simulink model "vehicle_ice"  (R2017a)
settings: Solver=FixedStepDiscrete  StartTime=0.0  StopTime=1400  FixedStep=abs(Ts)  RelTol=1e-3
InitFcn:
  | if ~exist('Ts')
  |     Ts = 1;
  | end
undefined symbols (not defined in the file or in its folder): elvio_cycle_nedc
libraries: elvio x10
settings Model: Creator=tstef  LastModifiedBy=elts2

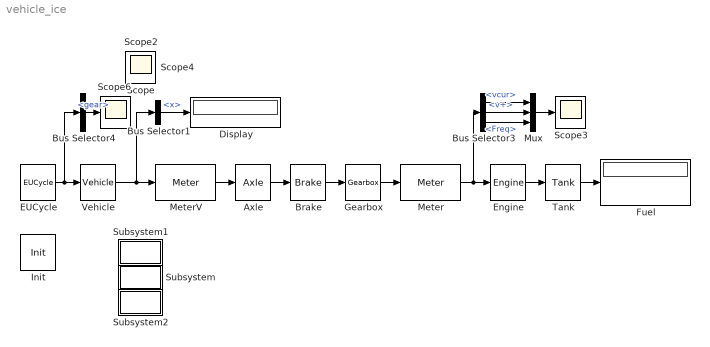
== system vehicle_ice ==
  Axle : elvio/Drive/Axle  radius=0.3  ratio=4  factor=0.1  FromTag1=Axle1  GotoTag1=MeterV1
  Brake : elvio/Drive/Brake  Tbrake=5000  FromTag1=Brake1  GotoTag1=Axle1
  Bus Selector1 : BusSelector  OutputSignals=info.x
  Bus Selector3 : BusSelector  OutputSignals=vcur,v+,Freq
  Bus Selector4 : BusSelector  OutputSignals=gear
  Display : Display
  EUCycle : elvio/Drive/EUCycle  data=elvio_cycle_nedc()
  Engine : elvio/Drive/Engine  Tmax=110  Tmin=0  Tfrict=12  Ploss=1000  lossf=1.1  lossnorm=500e3  lossR=0.2  FromTag1=Engine1  GotoTag1=Meter1
  Fuel : Display
  Gearbox : elvio/Drive/Gearbox  gears=[4 2.5 1.8 1.2 0.9 0.9]  factor=0.1  FromTag1=Gearbox1  GotoTag1=Brake1
  Init : elvio/Drive/Init  SystemSampleTime=-1
  Meter : elvio/Drive/Meter  FromTag1=Meter1  GotoTag1=Gearbox1
  MeterV : elvio/Drive/Meter  FromTag1=MeterV1  GotoTag1=Vehicle1
  Mux : Mux  Inputs=3
  Scope{,2..4,6} (5 alike) : Scope
      Scope4 mask Display: disp('1.484e+07')
  Subsystem : Subsystem
      settings: OpenFcn=elvio_plot_scatter(logsout);
      mask Display: disp('Scatter')
  Subsystem1 : Subsystem
      settings: OpenFcn=elvio_plot_energy(logsout);
      mask Display: disp('Energy')
  Subsystem2 : Subsystem
      settings: OpenFcn=elvio_plot_sources(logsout);
      mask Display: disp('Sources')
  Tank : elvio/Drive/Tank  GotoTag1=Engine1
  Vehicle : elvio/Drive/Vehicle  m=1200  Froll=150  Aeff=0.3:0.025:0.4  n=[1 5]  FromTag1=Vehicle1
  wires:
  Vehicle/1 -> MeterV/1, Bus Selector1/1
  Engine/1 -> Tank/1
  Tank/1 -> Fuel/1
  Gearbox/1 -> Meter/1
  Bus Selector1/1 -> Display/1  "<x>"
  MeterV/1 -> Axle/1
  Bus Selector3/3 -> Mux/3  "<Freq>"
  Bus Selector3/2 -> Mux/2  "<v+>"
  Mux/1 -> Scope3/1
  Meter/1 -> Bus Selector3/1, Engine/1
  Bus Selector3/1 -> Mux/1  "<vcur>"
  EUCycle/1 -> Bus Selector4/1, Vehicle/1
  Bus Selector4/1 -> Scope6/1  "<gear>"
  Axle/1 -> Brake/1
  Brake/1 -> Gearbox/1

== system vehicle_ice/Subsystem ==

== system vehicle_ice/Subsystem1 ==

== system vehicle_ice/Subsystem2 ==
